simulink model "single_fullbridge_PR"  (R2024a)
settings: Solver=FixedStepAuto  StartTime=0.0  StopTime=0.5  MaxStep=1e-7  MinStep=1e-8  RelTol=1e-3
libraries: spsMosfetLib x4, spsSeriesRLCBranchLib x3, spsCurrentMeasurementLib x2, spsDCVoltageSourceLib x1, spsTHDLib x1, spsTriangleGeneratorLib x1, spsVoltageMeasurementLib x1, sps_lib x1
settings Model: PacingRate=100000  Creator=Administrator  LastModifiedBy=Administrator

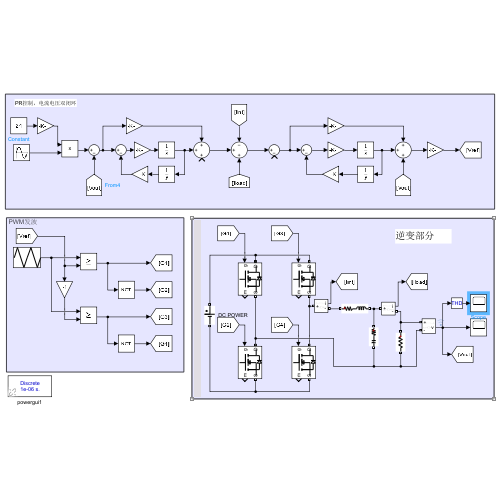
[thumbnail: Simulink's stored preview of the top-level diagram]
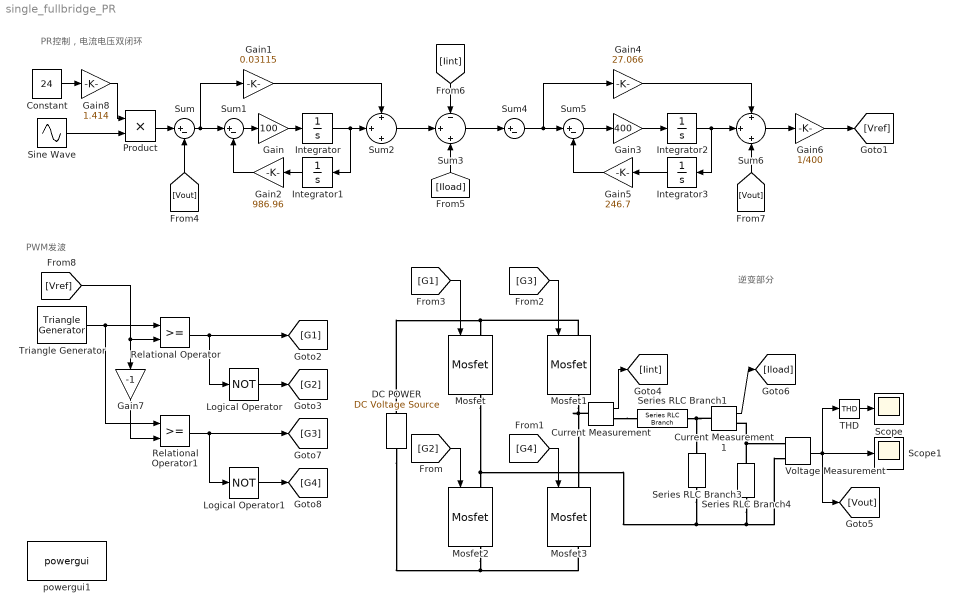
== system single_fullbridge_PR ==
  note: PR控制，电流电压双闭环
  note: PWM发波
  note: 逆变部分
  Constant : Constant  Value=24
  Current Measurement : spsCurrentMeasurementLib/Current Measurement  PhasorSimulation=off  OutputType=Complex  PSBequivalent=0
  Current Measurement1 : spsCurrentMeasurementLib/Current Measurement  PhasorSimulation=off  OutputType=Complex  PSBequivalent=0
  DC POWER : spsDCVoltageSourceLib/DC Voltage Source  Amplitude=48  Measurements=None
  Gain : Gain  Gain=100
  Gain1 : Gain  Gain=0.03115
  Gain2 : Gain  Gain=986.96
  Gain3 : Gain  Gain=400
  Gain4 : Gain  Gain=27.066
  Gain5 : Gain  Gain=246.7
  Gain6 : Gain  Gain=1/400
  Gain7 : Gain  Gain=-1
  Gain8 : Gain  Gain=1.414
  Integrator{,1..3} (4 alike) : Integrator
  Logical Operator : Logic  Operator=NOT  AllPortsSameDT=off  OutDataTypeStr=boolean
  Logical Operator1 : Logic  Operator=NOT  AllPortsSameDT=off  OutDataTypeStr=boolean
  Mosfet{,1..3} (4 alike) : spsMosfetLib/Mosfet  Ron=0.1  Lon=0  Rd=0.01  Vfd=0  IC=0  Rs=1e5  Cs=inf  Measurements=on
  Product : Product
  Relational Operator : RelationalOperator  OutDataTypeStr=boolean  RndMeth=Simplest  InputSameDT=off
  Relational Operator1 : RelationalOperator  OutDataTypeStr=boolean  RndMeth=Simplest  InputSameDT=off
  Scope : Scope
  Scope1 : Scope
  Series RLC Branch1 : spsSeriesRLCBranchLib/Series RLC Branch  LConnTagsString=__new0  RConnTagsString=__new0  BranchType=RL  Resistance=0.01  Inductance=4.06*1e-3  SetiL0=off  InitialCurrent=0  Capacitance=0  Setx0=off  InitialVoltage=0  Measurements=None
  Series RLC Branch3 : spsSeriesRLCBranchLib/Series RLC Branch  LConnTagsString=__new0  RConnTagsString=__new0  BranchType=RC  Resistance=0.01  Inductance=1e-3  SetiL0=off  InitialCurrent=0  Capacitance=1*1e-6  Setx0=off  InitialVoltage=0  Measurements=None
  Series RLC Branch4 : spsSeriesRLCBranchLib/Series RLC Branch  LConnTagsString=__new0  RConnTagsString=__new0  BranchType=R  Resistance=30  Inductance=1e-3  SetiL0=off  InitialCurrent=0  Capacitance=182.6*1e-3  Setx0=off  InitialVoltage=0  Measurements=None
  Sine Wave : Sin  Frequency=100*pi  SampleTime=0
  Sum{,1,4..5} (4 alike) : Sum  Inputs=|+-
  Sum2 : Sum  Inputs=+|+|+
  Sum3 : Sum  Inputs=-|+|+
  Sum6 : Sum  Inputs=+|+|+
  THD : spsTHDLib/THD  Freq=50  Ts=0
  Triangle Generator : spsTriangleGeneratorLib/Triangle Generator  Freq=1e4  Phase=90  Ts=0
  Voltage Measurement : spsVoltageMeasurementLib/Voltage Measurement  PhasorSimulation=off  OutputType=Complex  PSBequivalent=0
  powergui1 : sps_lib/powergui  Priority=1  SimulationMode=Discrete  SampleTime=1e-6  frequency=60  Iterations=50  frequencyindice=0  Pbase=100e6  ErrMax=1e-4  UnitsV=kV  UnitsW=MW  buscounter=0  FunctionMessages=off  echomessages=off  EnableUseOfTLC=off  CurrentSourceSwitches=off  DisableSnubberDevices=off  DisableRonSwitches=off  DisableVfSwitches=off  DisplayEquations=off  AutomaticDiscreteSolvers=off  SolverType=Tustin/Backward Euler (TBE)  Interpol=off  ExternalGateDelay=off  methode=off  Ts=100  x0status=blocks  SPID=on  SwTol=0  HookPort=off  NonlinearTolerance=1e-4  nMaxIteration=100  ContinueOnMaxIteration=off  RestoreLinks=warning  ResistiveCurrentMeasurement=off  Frange=[0:2:500]  Ylog=off  Xlog=on  ShowGrid=off  save=off  variable=ZData  structure=0  ZoomFFT=off  StartTime=0.0  cycles=1  DisplayStyle=1  fundamental=60  FreqAxis=off  MaxFrequency=1000  frequencyindicesteady=1  RmsSteady=1  display=off
  wires:
  THD/1 -> Scope/1
  Voltage Measurement/1 -> [Vout], Scope1/1, THD/1
  [G1] -> Mosfet/1
  [G3] -> Mosfet1/1
  [G4] -> Mosfet3/1
  [G2] -> Mosfet2/1
  Current Measurement/1 -> [Iint]
  Current Measurement1/1 -> [Iload]
  [Vout] -> Sum/2
  Sum/1 -> Gain1/1, Sum1/1
  Sum1/1 -> Gain/1
  Gain/1 -> Integrator/1
  Integrator/1 -> Integrator1/1, Sum2/2
  Integrator1/1 -> Gain2/1
  Gain2/1 -> Sum1/2
  Gain1/1 -> Sum2/1
  Sum3/1 -> Sum4/1
  [Iload] -> Sum3/3
  Sum2/1 -> Sum3/2
  [Iint] -> Sum3/1
  Gain3/1 -> Integrator2/1
  Gain5/1 -> Sum5/2
  Integrator2/1 -> Integrator3/1, Sum6/2
  Sum4/1 -> Gain4/1, Sum5/1
  Integrator3/1 -> Gain5/1
  Sum6/1 -> Gain6/1
  Gain4/1 -> Sum6/1
  Sum5/1 -> Gain3/1
  [Vout] -> Sum6/3
  Gain6/1 -> [Vref]
  Triangle Generator/1 -> Relational Operator1/1, Relational Operator/1
  [Vref] -> Relational Operator/2, Gain7/1
  Gain7/1 -> Relational Operator1/2
  Relational Operator/1 -> [G1], Logical Operator/1
  Relational Operator1/1 -> Logical Operator1/1, [G3]
  Logical Operator/1 -> [G2]
  Logical Operator1/1 -> [G4]
  Gain8/1 -> Product/1
  Sine Wave/1 -> Product/2
  Product/1 -> Sum/1
  Constant/1 -> Gain8/1
  connections:
  Mosfet/LConn1 -- DC POWER/RConn1 -- Mosfet1/LConn1
  Mosfet1/RConn1 -- Current Measurement/LConn1 -- Mosfet3/LConn1
  Mosfet3/RConn1 -- DC POWER/LConn1 -- Mosfet2/RConn1
  Mosfet2/LConn1 -- Mosfet/RConn1 -- Series RLC Branch3/RConn1 -- Series RLC Branch4/RConn1 -- Voltage Measurement/LConn2
  Series RLC Branch1/RConn1 -- Current Measurement1/LConn1 -- Series RLC Branch3/LConn1
  Current Measurement/RConn1 -- Series RLC Branch1/LConn1
  Series RLC Branch4/LConn1 -- Voltage Measurement/LConn1 -- Current Measurement1/RConn1
